simulink model "Lab1"  (R2018a)
settings: Solver=VariableStepAuto  StartTime=0.0  StopTime=10.0  RelTol=1e-3
settings Model: Creator=user  LastModifiedBy=user

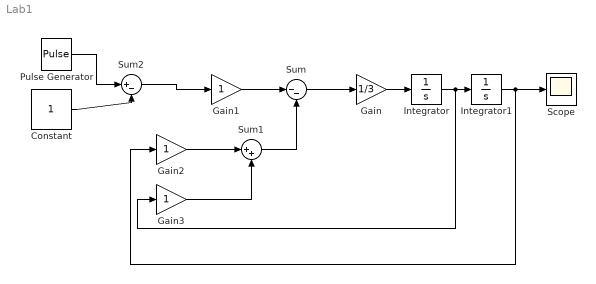
== system Lab1 ==
  Constant : Constant  VectorParams1D=off  SampleTime=-1
  Gain : Gain  Gain=1/3
  Gain1 : Gain
  Gain2 : Gain
  Gain3 : Gain
  Integrator : Integrator
  Integrator1 : Integrator
  Pulse Generator : DiscretePulseGenerator  PulseType=Time based  Amplitude=2  Period=10  PulseWidth=50
  Scope : Scope
  Sum : Sum  Inputs=|--
  Sum1 : Sum  Inputs=|++
  Sum2 : Sum  Inputs=|+-
  wires:
  Gain1/1 -> Sum/1
  Sum/1 -> Gain/1
  Sum1/1 -> Sum/2
  Gain2/1 -> Sum1/1
  Gain3/1 -> Sum1/2
  Gain/1 -> Integrator/1
  Integrator1/1 -> Scope/1, Gain2/1
  Integrator/1 -> Integrator1/1, Gain3/1
  Pulse Generator/1 -> Sum2/1
  Constant/1 -> Sum2/2
  Sum2/1 -> Gain1/1
